simulink model "Sensitivity_Analysis"  (R2023a)
settings: Solver=VariableStepAuto  StartTime=0.0  StopTime=10.0  RelTol=1e-3
undefined symbols (not defined in the file or in its folder): Ion, Lithium
libraries: spsSeriesRLCBranchLib x84, spsControlledCurrentSourceLib x54, spsCurrentMeasurementLib x42, spsVoltageMeasurementLib x42, spsControlledVoltageSourceLib x18, spsBatteryLib x6, sps_lib x6
(part 1 of 6)
settings Model: Creator=40485811  LastModifiedBy=40485811

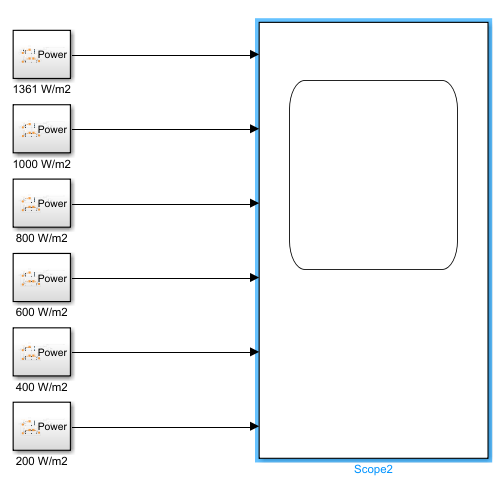
[thumbnail: Simulink's stored preview of the top-level diagram]
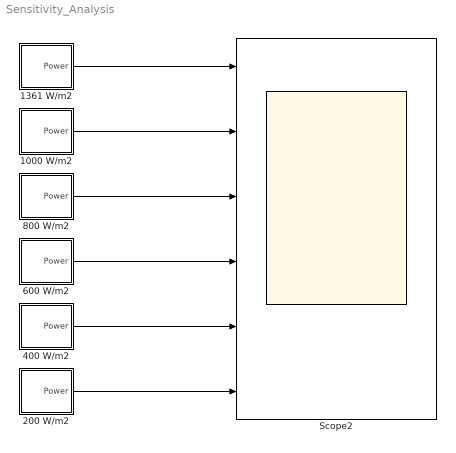
== system Sensitivity_Analysis ==
  1000 W/m2 : Subsystem
  1361 W/m2 : Subsystem
  200 W/m2 : Subsystem
  400 W/m2 : Subsystem
  600 W/m2 : Subsystem
  800 W/m2 : Subsystem
  Scope2 : Scope  NumInputPorts=6
  wires:
  1000 W/m2/1(Power) -> Scope2/2
  1361 W/m2/1(Power) -> Scope2/1
  800 W/m2/1(Power) -> Scope2/3
  600 W/m2/1(Power) -> Scope2/4
  200 W/m2/1(Power) -> Scope2/6
  400 W/m2/1(Power) -> Scope2/5

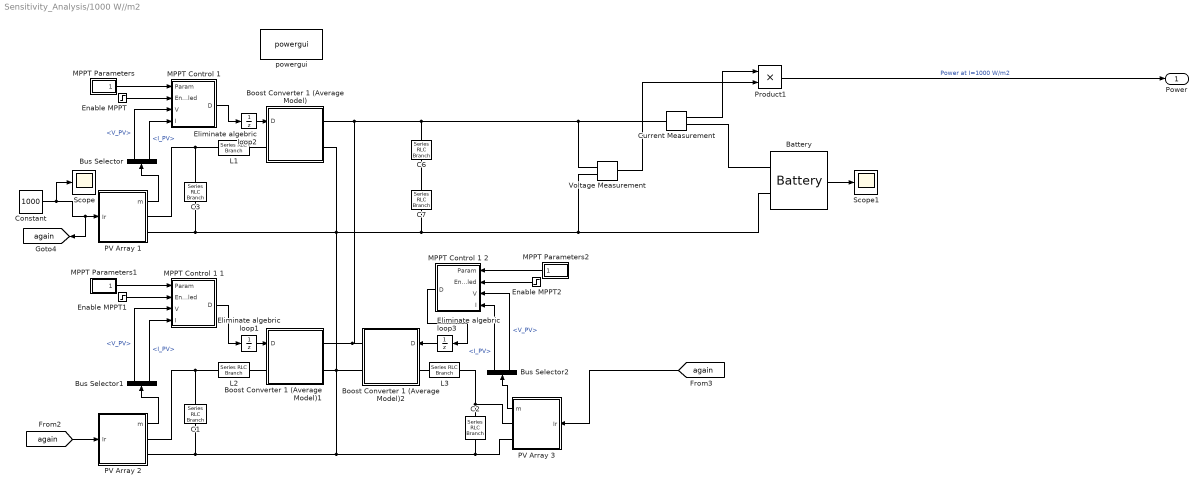
== system Sensitivity_Analysis/1000 W//m2 ==
  Battery : spsBatteryLib/Battery  BatType=Lithium-Ion  ShowTempParam=off  ThermalPreset=no  ShowAgeParam=off  NomV=7.2  NomQ=1000  SOC=100  Batt_Tr=30  PresetModel=on  MaxQ=1000  MinV=5.4  FullV=8.3807  Dis_rate=434.7826  R=7.2e-05  Normal_OP=904.3478  expZone="[7.77878      49.1304]"  current=[6.5 13 32.5]  Units=Time  Tci=20  NomT=20  T2=-30  MaxQ2=4.8  FullV2=7.1  Normal_OP2=5.655  expZone2="[6.58           1]"  Rca=0.6  ti=2000  Dp=0  Neq0=0  Tsim=1e6  Ta1=25  Qeol=5.4*0.9  Reol=0.013333*1.2  Char_age=[2.3478, 3]  Dis_age=[2.3478, 10]  N1=1500  N2=10500  N3=1000  N4=1400  Ta2=45  N5=950
  Boost Converter 1 (Average Model) : Subsystem  mask(Boost Converter (Average Model)){Ts=50e-6}
      mask prompts: Ts "Sample time:"
      mask Display: disp('Boost\n(Average)')
  Boost Converter 1 (Average Model)1 : Subsystem  mask(Boost Converter (Average Model)){Ts=50e-6}
      mask prompts: Ts "Sample time:"
      mask Display: disp('Boost\n(Average)')
  Boost Converter 1 (Average Model)2 : Subsystem  mask(Boost Converter (Average Model)){Ts=50e-6}
      mask prompts: Ts "Sample time:"
      mask Display: disp('Boost\n(Average)')
  Bus Selector : BusSelector  OutputSignals=V_PV,I_PV
  Bus Selector1 : BusSelector  OutputSignals=V_PV,I_PV
  Bus Selector2 : BusSelector  OutputSignals=V_PV,I_PV
  C1 : spsSeriesRLCBranchLib/Series RLC Branch  LConnTagsString=__new0  RConnTagsString=__new0  BranchType=C  Resistance=1.0  Inductance=1.0  SetiL0=off  InitialCurrent=0  Capacitance=100e-6  Setx0=off  InitialVoltage=0  Measurements=Branch voltage
  C2 : spsSeriesRLCBranchLib/Series RLC Branch  LConnTagsString=__new0  RConnTagsString=__new0  BranchType=C  Resistance=1.0  Inductance=1.0  SetiL0=off  InitialCurrent=0  Capacitance=100e-6  Setx0=off  InitialVoltage=0  Measurements=Branch voltage
  C3 : spsSeriesRLCBranchLib/Series RLC Branch  LConnTagsString=__new0  RConnTagsString=__new0  BranchType=C  Resistance=1.0  Inductance=1.0  SetiL0=off  InitialCurrent=0  Capacitance=100e-6  Setx0=off  InitialVoltage=0  Measurements=Branch voltage
  C6 : spsSeriesRLCBranchLib/Series RLC Branch  LConnTagsString=__new0  RConnTagsString=__new0  BranchType=C  Resistance=1.0  Inductance=1.0  SetiL0=off  InitialCurrent=0  Capacitance=24000e-06  Setx0=off  InitialVoltage=0  Measurements=None
  C7 : spsSeriesRLCBranchLib/Series RLC Branch  LConnTagsString=__new0  RConnTagsString=__new0  BranchType=C  Resistance=1.0  Inductance=1.0  SetiL0=off  InitialCurrent=0  Capacitance=24000e-06  Setx0=off  InitialVoltage=0  Measurements=None
  Constant : Constant  Value=1000
  Current Measurement : spsCurrentMeasurementLib/Current Measurement  PhasorSimulation=off  OutputType=Complex  PSBequivalent=0
  Eliminate algebric loop1 : UnitDelay  SampleTime=100e-6  HasFrameUpgradeWarning=on
  Eliminate algebric loop2 : UnitDelay  SampleTime=100e-6  HasFrameUpgradeWarning=on
  Eliminate algebric loop3 : UnitDelay  SampleTime=100e-6  HasFrameUpgradeWarning=on
  Enable MPPT : Step  Time=0.3  SampleTime=0
  Enable MPPT1 : Step  Time=0.3  SampleTime=0
  Enable MPPT2 : Step  Time=0.3  SampleTime=0
  L1 : spsSeriesRLCBranchLib/Series RLC Branch  LConnTagsString=__new0  RConnTagsString=__new0  BranchType=RL  Resistance=0.005  Inductance=5e-3  SetiL0=off  InitialCurrent=0  Capacitance=1e-6  Setx0=off  InitialVoltage=0  Measurements=None
  L2 : spsSeriesRLCBranchLib/Series RLC Branch  LConnTagsString=__new0  RConnTagsString=__new0  BranchType=RL  Resistance=0.005  Inductance=5e-3  SetiL0=off  InitialCurrent=0  Capacitance=1e-6  Setx0=off  InitialVoltage=0  Measurements=None
  L3 : spsSeriesRLCBranchLib/Series RLC Branch  LConnTagsString=__new0  RConnTagsString=__new0  BranchType=RL  Resistance=0.005  Inductance=5e-3  SetiL0=off  InitialCurrent=0  Capacitance=1e-6  Setx0=off  InitialVoltage=0  Measurements=None
  MPPT Parameters : Subsystem
  MPPT Parameters1 : Subsystem
  MPPT Parameters2 : Subsystem
  "MPPT Control 1 " : MATLAB Function  TreatAsAtomicUnit=on
  MPPT Control 1 1 : MATLAB Function  TreatAsAtomicUnit=on
  MPPT Control 1 2 : MATLAB Function  TreatAsAtomicUnit=on
  PV Array 1 : Subsystem  mask(PV array){ModuleType=SunPower SPR-305-WHT, Ncell=96, Nser=2500, Npar=2500, ModuleParameters=[ 64.2  5.96  54.7  5.58 ], ModelParameters=[ 0.037998  993.51  1.1753e-08  5.9602  1.3 ], Ts=50e-6, PlotVI_module=off, PlotVI_array=off}
      mask prompts: ModuleType "Module type:"; Ncell "Number of cells per module"; Nser "Number of series-connected  modules per string"; Npar "Number of parallel strings"; ModuleParameters "Module specifications under STC  [  Voc, Isc, Vmp, Imp ]"; ModelParameters "Model parameters for 1 module [ Rs, Rp, Isat, Iph, Qd ]"; Ts "Sample time"; PlotVI_module "Display  I-V and  P-V characteritics of one module"; PlotVI_array "Display  I-V and  P-V characteritics of array"
      mask help:
      | Model a PV array
      |
      | PV array consists of Npar strings of modules connected in parallel, each string consisting of Nser modules connected in series.
      |
      | The four PV model parameters (photo-generated current Iph, diode saturation current Isat, parallel resistance Rp and  series resistance Rs) are adjuted to fit the following four module characteristics measured under standard test conditions (STC : irradiance 1000 W/m^2, cell temperature=25 deg. C) and assuming a given "diode quality factor" (Qd) for the semiconductor:
      |   Voc = open circuit voltage
      |   Isc = short-circuit current
      |   Vmp,Imp = voltage and current at maximum power point
      |
      | Select a 'Module type' and then press Apply to see module parameters.
      | Note: Module characteristics are extracted from NREL System Advisor Model.
      mask init:
      | BlockName=gcb;
      | 
      | % SolarModuleSpec_Definition_v2.m
      | %================================
      | %
      | Type=1;
      | SolarModuleSpec(Type).Desc= 'Kyocera KD135GX-LP';
      | SolarModuleSpec(Type).nCells= 36;              % Number of cells in series
      | SolarModuleSpec(Type).Pmp= 135.044;            % Maximum power (W)
      | SolarModuleSpec(Type).Vmp= 17.7;               % Maximum power voltage (V) 
      | SolarModuleSpec(Type).Imp= 7.62959;            % Maximum power current (A)
      | SolarModuleSpec(Type).Voc= 22.0999;            % Open circuit voltage (V)
      | SolarModuleSpec(Type).Isc= 8.36955;            % Short circuit current (A)
      | SolarModuleSpec(Type).TempC_Pmp= -6.445e-001;  % Maximum power temp. coefficient (W/deg.C)
      | SolarModuleSpec(Type).TempC_Vmp= -8.200e-002;  % Maximum power voltage temp. coefficient (V/deg.C)
      | SolarModuleSpec(Type).TempC_Imp= -1.068e-003;  % Maximum power current temp. coefficient (A/deg.C
      | SolarModuleSpec(Type).TempC_Voc= -8.000e-002;  % Open circuit voltage temp. coefficient (V/deg.C)
      | SolarModuleSpec(Type).TempC_Isc= 5.022e-003;   % Short circuit current temp. coefficient (A/deg.C)
      | SolarModuleSpec(Type).Rs= 0.10593;             % Series resistance of PV model (ohms)
      | SolarModuleSpec(Type).Rp= 142.84;              % Parallel resistance of PV model (ohms)
      | SolarModuleSpec(Type).Isat= 9.845e-07;         % Diode saturation current of PV model (A)
      | SolarModuleSpec(Type).Iph=  8.3758;            % Light-generated photo-current  of PV model (A)
      | SolarModuleSpec(Type).Qd= 1.5;                 % Diode quality factor of PV model
      | %-------------------------------------------------------------------------
      | %
      | Type=2;
      | SolarModuleSpec(Type).Desc= 'Kyocera KD205GX-LP';
      | SolarModuleSpec(Type).nCells= 54;              % Number of cells in series
      | SolarModuleSpec(Type).Pmp= 205.075;            % Maximum power (W)
      | SolarModuleSpec(Type).Vmp= 26.6;               % Maximum power voltage (V) 
      | SolarModuleSpec(Type).Imp= 7.70959;            % Maximum power current (A)
      | SolarModuleSpec(Type).Voc= 33.1999;            % Open circuit voltage (V)
      | SolarModuleSpec(Type).Isc= 8.35955;            % Short circuit current (A)
      | SolarModuleSpec(Type).TempC_Pmp= -9.770e-001;  % Maximum power temp. coefficient (W/deg.C)
      | SolarModuleSpec(Type).TempC_Vmp= -1.230e-001;  % Maximum power voltage temp. coefficient (V/deg.C)
      | SolarModuleSpec(Type).TempC_Imp= -1.079e-003;  % Maximum power current temp. coefficient (A/deg.C
      | SolarModuleSpec(Type).TempC_Voc= -1.200e-001;  % Open circuit voltage temp. coefficient (V/deg.C)
      | SolarModuleSpec(Type).TempC_Isc= 5.016e-003;   % Short circuit current temp. coefficient (A/deg.C)
      | SolarModuleSpec(Type).Rs= 0.15945;             % Series resistance of PV model (ohms)
      | SolarModuleSpec(Type).Rp= 1010.6;              % Parallel resistance of PV model (ohms)
      | SolarModuleSpec(Type).Isat=  9.7399e-07;       % Diode saturation current of PV model (A)
      | SolarModuleSpec(Type).Iph= 8.3642;             % Light-generated photo-current  of PV model (A)
      | SolarModuleSpec(Type).Qd= 1.5;                 % Diode quality factor of PV model
      | %-------------------------------------------------------------------------
      | %
      | Type=3;
      | SolarModuleSpec(Type).Desc= 'Mitsubishi PV-UD190MF5';
      | SolarModuleSpec(Type).nCells= 50;              % Number of cells in series
      | SolarModuleSpec(Type).Pmp= 190.503;            % Maximum power (W)
      | SolarModuleSpec(Type).Vmp= 24.6999;            % Maximum power voltage (V) 
      | SolarModuleSpec(Type).Imp= 7.71272;            % Maximum power current (A)
      | SolarModuleSpec(Type).Voc= 30.8006;            % Open circuit voltage (V)
      | SolarModuleSpec(Type).Isc= 8.23289;            % Short circuit current (A)
      | SolarModuleSpec(Type).TempC_Pmp= -8.597e-001;  % Maximum power temp. coefficient (W/deg.C)
      | SolarModuleSpec(Type).TempC_Vmp= -1.090e-001;  % Maximum power voltage temp. coefficient (V/deg.C)
      | SolarModuleSpec(Type).TempC_Imp= -7.713e-004;  % Maximum power current temp. coefficient (A/deg.C
      | SolarModuleSpec(Type).TempC_Voc= -1.050e-001;  % Open circuit voltage temp. coefficient (V/deg.C)
      | SolarModuleSpec(Type).TempC_Isc= 4.446e-003;   % Short circuit current temp. coefficient (A/deg.C)
      | SolarModuleSpec(Type).Rs= 0.20758;             % Series resistance of PV model (ohms)
      | SolarModuleSpec(Type).Rp= 975.6;               % Parallel resistance of PV model (ohms)
      | SolarModuleSpec(Type).Isat= 7.9676e-08;        % Diode saturation current of PV model (A)
      | SolarModuleSpec(Type).Iph= 8.2649;             % Light-generated photo-current  of PV model (A)
      | SolarModuleSpec(Type).Qd= 1.3;                 % Diode quality factor of PV model
      | %-------------------------------------------------------------------------
      | %
      | Type=4;
      | SolarModuleSpec(Type).Desc= 'Sanyo HIP-225HDE1';
      | SolarModuleSpec(Type).nCells= 60;              % Number of cells in series
      | SolarModuleSpec(Type).Pmp= 224.899;            % Maximum power (W)
      | SolarModuleSpec(Type).Vmp= 33.9;               % Maximum power voltage (V) 
      | SolarModuleSpec(Type).Imp= 6.63419;            % Maximum power current (A)
      | SolarModuleSpec(Type).Voc= 41.7984;            % Open circuit voltage (V)
      | SolarModuleSpec(Type).Isc= 7.13383;            % Short circuit current (A)
      | SolarModuleSpec(Type).TempC_Pmp= -6.925e-001;  % Maximum power temp. coefficient (W/deg.C)
      | SolarModuleSpec(Type).TempC_Vmp= -1.010e-001;  % Maximum power voltage temp. coefficient (V/deg.C)
      | SolarModuleSpec(Type).TempC_Imp= -6.634e-004;  % Maximum power current temp. coefficient (A/deg.C
      | SolarModuleSpec(Type).TempC_Voc= -1.050e-001;  % Open circuit voltage temp. coefficient (V/deg.C)
      | SolarModuleSpec(Type).TempC_Isc= 2.140e-003;   % Short circuit current temp. coefficient (A/deg.C)
      | SolarModuleSpec(Type).Rs=  0.20439;            % Series resistance of PV model (ohms)
      | SolarModuleSpec(Type).Rp= 1830.7;              % Parallel resistance of PV model (ohms)
      | SolarModuleSpec(Type).Isat=  3.0815e-07;       % Diode saturation current of PV model (A)
      | SolarModuleSpec(Type).Iph=  7.145;             % Light-generated photo-current  of PV model (A)
      | SolarModuleSpec(Type).Qd= 1.6;                 % Diode quality factor of PV model
      | %-------------------------------------------------------------------------
      | %
      | 
      | Type=5;
      | % NREL : 2007(E)
      | SolarModuleSpec(Type).Desc= 'SunPower SPR-305-WHT';
      | SolarModuleSpec(Type).nCells= 96;              % Number of cells in series
      | SolarModuleSpec(Type).Pmp= 305.2;              % Maximum power (W)
      | SolarModuleSpec(Type).Vmp= 54.70;              % Maximum power voltage (V) 
      | SolarModuleSpec(Type).Imp= 5.58;               % Maximum power current (A)
      | SolarModuleSpec(Type).Voc= 64.20;              % Open circuit voltage (V)
      | SolarModuleSpec(Type).Isc= 5.96;               % Short circuit current (A)
      | SolarModuleSpec(Type).TempC_Pmp= -1.154e+000;  % Maximum power temp. coefficient (W/deg.C)
      | SolarModuleSpec(Type).TempC_Vmp= -1.860e-001;  % Maximum power voltage temp. coefficient (V/deg.C)
      | SolarModuleSpec(Type).TempC_Imp= -2.120e-003;  % Maximum power current temp. coefficient (A/deg.C
      | SolarModuleSpec(Type).TempC_Voc= -1.770e-001;  % Open circuit voltage temp. coefficient (V/deg.C)
      | SolarModuleSpec(Type).TempC_Isc= 3.516e-003;   % Short circuit current temp. coefficient (A/deg.C)
      | SolarModuleSpec(Type).Rs= 0.037998;            % Series resistance of PV model (ohms)
      | SolarModuleSpec(Type).Rp= 993.51;              % Parallel resistance of PV model (ohms)
      | SolarModuleSpec(Type).Isat= 1.1753e-08;        % Diode saturation current of PV model (A)
      | SolarModuleSpec(Type).Iph= 5.9602;             % Light-generated photo-current  of PV model (A)
      | SolarModuleSpec(Type).Qd= 1.3;                 % Diode quality factor of PV model
      | %-------------------------------------------------------------------------
      | %
      | Type=6;
      | SolarModuleSpec(Type).Desc= 'Suntech STP270S-24_Vb';
      | SolarModuleSpec(Type).nCells= 72;              % Number of cells in series
      | SolarModuleSpec(Type).Pmp= 269.843;            % Maximum power (W)
      | SolarModuleSpec(Type).Vmp= 35;                 % Maximum power voltage (V) 
      | SolarModuleSpec(Type).Imp= 7.70979;            % Maximum power current (A)
      | SolarModuleSpec(Type).Voc= 44.4999;            % Open circuit voltage (V)
      | SolarModuleSpec(Type).Isc= 8.19978;            % Short circuit current (A)
      | SolarModuleSpec(Type).TempC_Pmp= -1.204e+000;  % Maximum power temp. coefficient (W/deg.C)
      | SolarModuleSpec(Type).TempC_Vmp= -1.567e-001;  % Maximum power voltage temp. coefficient (V/deg.C)
      | SolarModuleSpec(Type).TempC_Imp= 1.234e-004;   % Maximum power current temp. coefficient (A/deg.C
      | SolarModuleSpec(Type).TempC_Voc= -1.504e-001;  % Open circuit voltage temp. coefficient (V/deg.C)
      | SolarModuleSpec(Type).TempC_Isc= 4.969e-003;   % Short circuit current temp. coefficient (A/deg.C)
      | SolarModuleSpec(Type).Rs= 0.32025;             % Series resistance of PV model (ohms)
      | SolarModuleSpec(Type).Rp= 2562.3;              % Parallel resistance of PV model (ohms)
      | SolarModuleSpec(Type).Isat= 8.8992e-07;        % Diode saturation current of PV model (A)
      | SolarModuleSpec(Type).Iph= 8.2979;             % Light-generated photo-current  of PV model (A)
      | SolarModuleSpec(Type).Qd= 1.5;                 % Diode quality factor of PV model
      | % 
      | %-------------------------------------------------------------------------
      | %
      | Type=7;
      | SolarModuleSpec(Type).Desc= 'Canadian Solar CS5P-220M';
      | SolarModuleSpec(Type).nCells= 96;              % Number of cells in series
      | SolarModuleSpec(Type).Pmp= 219.72;             % Maximum power (W)
      | SolarModuleSpec(Type).Vmp= 48.3159;            % Maximum power voltage (V) 
      | SolarModuleSpec(Type).Imp= 4.54758;            % Maximum power current (A)
      | SolarModuleSpec(Type).Voc= 59.2618;            % Open circuit voltage (V)
      | SolarModuleSpec(Type).Isc= 5.09261;            % Short circuit current (A)
      | SolarModuleSpec(Type).TempC_Pmp= -1.031e+000;  % Maximum power temp. coefficient (W/deg.C)
      | SolarModuleSpec(Type).TempC_Vmp= -2.355e-001;  % Maximum power voltage temp. coefficient (V/deg.C)
      | SolarModuleSpec(Type).TempC_Imp= 8.231e-004;   % Maximum power current temp. coefficient (A/deg.C
      | SolarModuleSpec(Type).TempC_Voc= -2.170e-001;  % Open circuit voltage temp. coefficient (V/deg.C)
      | SolarModuleSpec(Type).TempC_Isc= 2.022e-003;   % Short circuit current temp. coefficient (A/deg.C)
      | SolarModuleSpec(Type).Rs= 0.24807;             % Series resistance of PV model (ohms)
      | SolarModuleSpec(Type).Rp= 235.76;              % Parallel resistance of PV model (ohms)
      | SolarModuleSpec(Type).Isat= 5.3103e-07;        % Diode saturation current of PV model (A)
      | SolarModuleSpec(Type).Iph= 5.098;              % Light-generated photo-current  of PV model (A)
      | SolarModuleSpec(Type).Qd= 1.5;                 % Diode quality factor of PV model
      | %-------------------------------------------------------------------------
      | %
      | Type=8;
      | SolarModuleSpec(Type).Desc= 'BP Solar SX3190';
      | SolarModuleSpec(Type).nCells= 50;              % Number of cells in series
      | SolarModuleSpec(Type).Pmp= 190.258;            % Maximum power (W)
      | SolarModuleSpec(Type).Vmp= 24.3003;            % Maximum power voltage (V) 
      | SolarModuleSpec(Type).Imp= 7.82945;            % Maximum power current (A)
      | SolarModuleSpec(Type).Voc= 30.6021;            % Open circuit voltage (V)
      | SolarModuleSpec(Type).Isc= 8.51029;            % Short circuit current (A)
      | SolarModuleSpec(Type).TempC_Pmp= -9.306e-001;  % Maximum power temp. coefficient (W/deg.C)
      | SolarModuleSpec(Type).TempC_Vmp= -1.140e-001;  % Maximum power voltage temp. coefficient (V/deg.C)
      | SolarModuleSpec(Type).TempC_Imp= -1.566e-003;  % Maximum power current temp. coefficient (A/deg.C
      | SolarModuleSpec(Type).TempC_Voc= -1.110e-001;  % Open circuit voltage temp. coefficient (V/deg.C)
      | SolarModuleSpec(Type).TempC_Isc= 5.532e-003;   % Short circuit current temp. coefficient (A/deg.C)
      | SolarModuleSpec(Type).Rs= 0.17514;             % Series resistance of PV model (ohms)
      | SolarModuleSpec(Type).Rp= 755.51;              % Parallel resistance of PV model (ohms)
      | SolarModuleSpec(Type).Isat= 1.0647e-06;       % Diode saturation current of PV model (A)
      | SolarModuleSpec(Type).Iph= 8.5158;             % Light-generated photo-current  of PV model (A)
      | SolarModuleSpec(Type).Qd= 1.5;                 % Diode quality factor of PV model
      | %-------------------------------------------------------------------------
      | %
      | Type=9;
      | SolarModuleSpec(Type).Desc= 'First Solar FS-272';
      | SolarModuleSpec(Type).nCells= 116;             % Number of cells in series
      | SolarModuleSpec(Type).Pmp= 71.326;             % Maximum power (W)
      | SolarModuleSpec(Type).Vmp= 70.558;             % Maximum power voltage (V) 
      | SolarModuleSpec(Type).Imp= 1.01088;            % Maximum power current (A)
      | SolarModuleSpec(Type).Voc= 94.5738;            % Open circuit voltage (V)
      | SolarModuleSpec(Type).Isc= 1.18103;            % Short circuit current (A)
      | SolarModuleSpec(Type).TempC_Pmp= -2.332e-001;  % Maximum power temp. coefficient (W/deg.C)
      | SolarModuleSpec(Type).TempC_Vmp= -2.060e-001;  % Maximum power voltage temp. coefficient (V/deg.C)
      | SolarModuleSpec(Type).TempC_Imp= -3.538e-004;  % Maximum power current temp. coefficient (A/deg.C
      | SolarModuleSpec(Type).TempC_Voc= -2.690e-001;  % Open circuit voltage temp. coefficient (V/deg.C)
      | SolarModuleSpec(Type).TempC_Isc= 5.433e-004;   % Short circuit current temp. coefficient (A/deg.C)
      | SolarModuleSpec(Type).Rs= 7.7692;              % Series resistance of PV model (ohms)
      | SolarModuleSpec(Type).Rp= 1044.9;              % Parallel resistance of PV model (ohms)
      | SolarModuleSpec(Type).Isat= 1.1116e-068;       % Diode saturation current of PV model (A)
      | SolarModuleSpec(Type).Iph= 1.1898;             % Light-generated photo-current  of PV model (A)
      | SolarModuleSpec(Type).Qd= 2.3;                 % Diode quality factor of PV model
      | %-------------------------------------------------------------------------
      | %
      | Type=10;
      | SolarModuleSpec(Type).Desc= 'SunPower 128-cell Module';
      | SolarModuleSpec(Type).nCells= 128;             % Number of cells in series
      | SolarModuleSpec(Type).Pmp= 400.048;            % Maximum power (W)
      | SolarModuleSpec(Type).Vmp= 72.8992;            % Maximum power voltage (V) 
      | SolarModuleSpec(Type).Imp= 5.48769;            % Maximum power current (A)
      | SolarModuleSpec(Type).Voc= 85.2983;            % Open circuit voltage (V)
      | SolarModuleSpec(Type).Isc= 5.8675;             % Short circuit current (A)
      | SolarModuleSpec(Type).TempC_Pmp= -1.638e+000;  % Maximum power temp. coefficient (W/deg.C)
      | SolarModuleSpec(Type).TempC_Vmp= -2.760e-001;  % Maximum power voltage temp. coefficient (V/deg.C)
      | SolarModuleSpec(Type).TempC_Imp= -1.690e-003;  % Maximum power current temp. coefficient (A/deg.C
      | SolarModuleSpec(Type).TempC_Voc= -2.664e-001;  % Open circuit voltage temp. coefficient (V/deg.C)
      | SolarModuleSpec(Type).TempC_Isc= 1.837e-003;   % Short circuit current temp. coefficient (A/deg.C)
      | SolarModuleSpec(Type).Rs= 0.12264;             % Series resistance of PV model (ohms)
      | SolarModuleSpec(Type).Rp= 859.93;              % Parallel resistance of PV model (ohms)
      | SolarModuleSpec(Type).Isat= 2.3385e-09;        % Diode saturation current of PV model (A)
      | SolarModuleSpec(Type).Iph= 5.8683;             % Light-generated photo-current  of PV model (A)
      | SolarModuleSpec(Type).Qd= 1.2;                 % Diode quality factor of PV model
      | %-------------------------------------------------------------------------
      | 
      | Type=strmatch(ModuleType,char(SolarModuleSpec.Desc));
      | 
      | k= 1.3806e-23; % Boltzman constant (J.K^-1)
      | q=1.6022e-19;  % electron charge  (C)
      | T=273+25;
      | 
      | nCells=SolarModuleSpec(Type).nCells;
      | Voc=SolarModuleSpec(Type).Voc;
      | Isc=SolarModuleSpec(Type).Isc;
      | Vm=SolarModuleSpec(Type).Vmp;
      | Im=SolarModuleSpec(Type).Imp;
      | 
      | set_param(BlockName,'Ncell',num2str(nCells));
      | str=sprintf('[ %g  %g  %g  %g ]',Voc,Isc,Vm,Im);
      | set_param(BlockName,'ModuleParameters',str);
      | 
      | Rs=SolarModuleSpec(Type).Rs;
      | Rp=SolarModuleSpec(Type).Rp; 
      | Isat=SolarModuleSpec(Type).Isat;
      | Iph=SolarModuleSpec(Type).Iph;            
      | Qd=SolarModuleSpec(Type).Qd;
      | 
      | VT=k*T/q*nCells*Qd;
      | 
      | str=sprintf('[ %g  %g  %g  %g  %g ]',Rs,Rp,Isat,Iph, Qd);
      | set_param(BlockName,'ModelParameters',str)
      | 
      | Iph_array=Iph*Npar;
      | Isat_array=Isat*Npar;
      | VT_array=VT*Nser;
      | Rs_array=Rs*Nser/Npar;
      | Rp_array=Rp*Nser/Npar;
      | %
      | %% Plot I-V & P-V characteristics of one module
      | %==============================================
      | if PlotVI_module | PlotVI_array
      |     assignin('base','Voc',Voc);
      |     assignin('base','Isc',Isc);
      |     assignin('base','Rs',Rs);
      |     assignin('base','Rp',Rp);
      |     assignin('base','Isat',Isat);
      |     assignin('base','VT',VT);
      |      
      |     if PlotVI_module, 
      |         F1=figure('Name','I-V and P-V characteristics of one module at 25 deg.C');
      |     end
      |     if PlotVI_array ,
      |         F2=figure('Name','I-V and P-V characteristics of array at 25 deg.C');  
      |     end
      |     load_system('PV_model_Param');
      |     
      |     for ksun=1:-0.25:0.25
      |         assignin('base','Iph',Iph*ksun)
      |         sim('PV_model_Param');
      |         n=find(I_PV>=0);
      |         I_PV=I_PV(n);
      |         V_PV=V_PV(n);
      |         P_PV=V_PV.*I_PV;
      |         
      |         if PlotVI_module
      |             figure(F1);
      |             subplot(211)
      |             if ksun==1
      |                 plot(V_PV,I_PV,'b',[0  Vm Voc], [Isc Im 0],'ro')
      |                 text(Voc/15,Isc*1.1,'1 kW/m^2')
      |                 hold on
      |                 grid
      |             else
      |                 plot(V_PV,I_PV,'--m')
      |                 text(Voc/15, Isc*(ksun+0.1) , sprintf('%g kW/m^2',ksun))
      |             end
      | 
      |             subplot(212) 
      |             if ksun==1
      |                 plot(V_PV,P_PV,'b',[0  Vm Voc], [0 Im*Vm 0],'ro')
      |                 text(Vm*1.02,Vm*Im,'1 kW/m^2')
      |                 hold on
      |                 grid
      |             else
      |                 n= find(P_PV==max(P_PV));
      |                 plot(V_PV,P_PV,'--m', V_PV(n) , P_PV(n),'mo')
      |                 text(Vm*1.02, Vm*Im*ksun, sprintf('%g kW/m^2',ksun))
      |             end
      |             subplot(211)
      |             ylabel('Current (A)')
      |             xlabel('Voltage (V)')
      |             title(sprintf('Module type: %s',SolarModuleSpec(Type).Desc))
      |             axis_xy=axis;
      |             axis_xy(4)=Isc*1.2;
      |             axis(axis_xy);
      |             
      |             subplot(212)
      |             ylabel('Power (W)')
      |             xlabel('Voltage (V)')
      |             axis_xy=axis;
      |             axis_xy(4)=Vm*Im*1.2;
      |             axis(axis_xy);
      |                   
      |             set_param(BlockName,'PlotVI_module', 'off')
      |         end
      |         
      |         if PlotVI_array
      |             figure(F2);
      |             subplot(211)
      |             if ksun==1
      |                 plot(V_PV*Nser,I_PV*Npar,'b',[0  Vm Voc]*Nser, [Isc Im 0]*Npar,'ro')
      |                 text(Voc/15*Nser,Isc*1.1*Npar,'1 kW/m^2')
      |                 hold on
      |                 grid
      |             else
      |                 plot(V_PV*Nser,I_PV*Npar,'--m')
      |                 text(Voc*Nser/15, Isc*Npar*(ksun+0.1) , sprintf('%g kW/m^2',ksun))
      |             end
      |            
      | 
      |             subplot(212)
      |             if ksun==1
      |                 plot(V_PV*Nser,P_PV*Nser*Npar,'b',[0  Vm Voc]*Nser, [0 Im*Vm 0]*Nser*Npar,'ro')
      |                 text(Vm*Nser*1.02,Vm*Im*Nser*Npar,'1 kW/m^2')
      |                 hold on
      |                 grid
      |             else
      |                 n= find(P_PV==max(P_PV));
      |                 plot(V_PV*Nser,P_PV*Nser*Npar,'--m', V_PV(n)*Nser , P_PV(n)*Nser*Npar,'mo')
      |                 text(Vm*Nser*1.02, Vm*Im*Nser*Npar*ksun, sprintf('%g kW/m^2',ksun))
      |             end 
      |             subplot(211)
      |             ylabel('Current (A)')
      |             xlabel('Voltage (V)')
      |             title(sprintf('Array type: %s; %d series modules; %d parallel strings',SolarModuleSpec(Type).Desc,Nser,Npar));
      |             axis_xy=axis;
      |             axis_xy(4)=Isc*Npar*1.2;
      |             axis(axis_xy);
      |             
      |             subplot(212)
      |             ylabel('Power (W)')
      |             xlabel('Voltage (V)')
      |             xis_xy=axis;
      |             axis_xy(4)=Vm*Im*Nser*Npar*1.2;
      |             axis(axis_xy);
      |             
      |             set_param(BlockName,'PlotVI_array', 'off')
      |         end
      |         
      |     end  
      | end
      mask TypeOptions ModuleType: BP Solar SX3190 | Canadian Solar CS5P-220M | First Solar FS-272 | Kyocera KD135GX-LP | Kyocera KD205GX-LP | Mitsubishi PV-UD190MF5 | Sanyo HIP-225HDE1 | SunPower SPR-305-WHT | SunPower SPR-400-WHT | Suntech STP270S-24_Vb
      mask Display: image(imread('panel.jpg'))
  PV Array 2 : Subsystem  mask(PV array){ModuleType=SunPower SPR-305-WHT, Ncell=96, Nser=2500, Npar=2500, ModuleParameters=[ 64.2  5.96  54.7  5.58 ], ModelParameters=[ 0.037998  993.51  1.1753e-08  5.9602  1.3 ], Ts=50e-6, PlotVI_module=off, PlotVI_array=off}
      mask prompts: ModuleType "Module type:"; Ncell "Number of cells per module"; Nser "Number of series-connected  modules per string"; Npar "Number of parallel strings"; ModuleParameters "Module specifications under STC  [  Voc, Isc, Vmp, Imp ]"; ModelParameters "Model parameters for 1 module [ Rs, Rp, Isat, Iph, Qd ]"; Ts "Sample time"; PlotVI_module "Display  I-V and  P-V characteritics of one module"; PlotVI_array "Display  I-V and  P-V characteritics of array"
      mask help:
      | Model a PV array
      |
      | PV array consists of Npar strings of modules connected in parallel, each string consisting of Nser modules connected in series.
      |
      | The four PV model parameters (photo-generated current Iph, diode saturation current Isat, parallel resistance Rp and  series resistance Rs) are adjuted to fit the following four module characteristics measured under standard test conditions (STC : irradiance 1000 W/m^2, cell temperature=25 deg. C) and assuming a given "diode quality factor" (Qd) for the semiconductor:
      |   Voc = open circuit voltage
      |   Isc = short-circuit current
      |   Vmp,Imp = voltage and current at maximum power point
      |
      | Select a 'Module type' and then press Apply to see module parameters.
      | Note: Module characteristics are extracted from NREL System Advisor Model.
      mask init: same as Sensitivity_Analysis/1000 W//m2/PV Array 1
      mask TypeOptions ModuleType: BP Solar SX3190 | Canadian Solar CS5P-220M | First Solar FS-272 | Kyocera KD135GX-LP | Kyocera KD205GX-LP | Mitsubishi PV-UD190MF5 | Sanyo HIP-225HDE1 | SunPower SPR-305-WHT | SunPower SPR-400-WHT | Suntech STP270S-24_Vb
      mask Display: image(imread('panel.jpg'))
  PV Array 3 : Subsystem  mask(PV array){ModuleType=SunPower SPR-305-WHT, Ncell=96, Nser=2500, Npar=2500, ModuleParameters=[ 64.2  5.96  54.7  5.58 ], ModelParameters=[ 0.037998  993.51  1.1753e-08  5.9602  1.3 ], Ts=50e-6, PlotVI_module=off, PlotVI_array=off}
      mask prompts: ModuleType "Module type:"; Ncell "Number of cells per module"; Nser "Number of series-connected  modules per string"; Npar "Number of parallel strings"; ModuleParameters "Module specifications under STC  [  Voc, Isc, Vmp, Imp ]"; ModelParameters "Model parameters for 1 module [ Rs, Rp, Isat, Iph, Qd ]"; Ts "Sample time"; PlotVI_module "Display  I-V and  P-V characteritics of one module"; PlotVI_array "Display  I-V and  P-V characteritics of array"
      mask help:
      | Model a PV array
      |
      | PV array consists of Npar strings of modules connected in parallel, each string consisting of Nser modules connected in series.
      |
      | The four PV model parameters (photo-generated current Iph, diode saturation current Isat, parallel resistance Rp and  series resistance Rs) are adjuted to fit the following four module characteristics measured under standard test conditions (STC : irradiance 1000 W/m^2, cell temperature=25 deg. C) and assuming a given "diode quality factor" (Qd) for the semiconductor:
      |   Voc = open circuit voltage
      |   Isc = short-circuit current
      |   Vmp,Imp = voltage and current at maximum power point
      |
      | Select a 'Module type' and then press Apply to see module parameters.
      | Note: Module characteristics are extracted from NREL System Advisor Model.
      mask init: same as Sensitivity_Analysis/1000 W//m2/PV Array 1
      mask TypeOptions ModuleType: BP Solar SX3190 | Canadian Solar CS5P-220M | First Solar FS-272 | Kyocera KD135GX-LP | Kyocera KD205GX-LP | Mitsubishi PV-UD190MF5 | Sanyo HIP-225HDE1 | SunPower SPR-305-WHT | SunPower SPR-400-WHT | Suntech STP270S-24_Vb
      mask Display: image(imread('panel.jpg'))
  Product1 : Product
  Scope : Scope
  Scope1 : Scope
  Voltage Measurement : spsVoltageMeasurementLib/Voltage Measurement  PhasorSimulation=off  OutputType=Complex  PSBequivalent=0
  powergui : sps_lib/powergui  Priority=1  SimulationMode=Continuous  SampleTime=50e-6  frequency=60  Iterations=50  frequencyindice=0  Pbase=100e6  ErrMax=1e-4  UnitsV=kV  UnitsW=MW  buscounter=0  FunctionMessages=off  echomessages=off  EnableUseOfTLC=off  CurrentSourceSwitches=off  DisableSnubberDevices=off  DisableRonSwitches=off  DisableVfSwitches=off  DisplayEquations=off  AutomaticDiscreteSolvers=off  SolverType=Tustin/Backward Euler (TBE)  Interpol=off  ExternalGateDelay=off  methode=off  Ts=100  x0status=blocks  SPID=on  SwTol=0  HookPort=off  NonlinearTolerance=1e-4  nMaxIteration=100  ContinueOnMaxIteration=off  RestoreLinks=warning  ResistiveCurrentMeasurement=off  Frange=[0:2:500]  Ylog=off  Xlog=on  ShowGrid=off  save=off  variable=ZData  structure=0  ZoomFFT=off  StartTime=0.0  cycles=1  DisplayStyle=1  fundamental=60  FreqAxis=off  MaxFrequency=1000  frequencyindicesteady=1  RmsSteady=1  display=off
  Power : Outport
  tag scope: again=global
  wires:
  Constant/1 -> PV Array 1/1(Ir), [again], Scope/1
  Bus Selector1/1 -> MPPT Control 1 1/3(V)  "<V_PV>"
  Enable MPPT/1 -> "MPPT Control 1 "/2(Enabled)
  Enable MPPT2/1 -> MPPT Control 1 2/2(Enabled)
  Eliminate algebric loop1/1 -> Boost Converter 1 (Average Model)1/1(D)
  Bus Selector1/2 -> MPPT Control 1 1/4(I)  "<I_PV>"
  Bus Selector2/2 -> MPPT Control 1 2/4(I)  "<I_PV>"
  Bus Selector/2 -> "MPPT Control 1 "/4(I)  "<I_PV>"
  PV Array 1/1(m) -> Bus Selector/1
  MPPT Parameters2/1(Param) -> MPPT Control 1 2/1(Param)
  "MPPT Control 1 "/1(D) -> Eliminate algebric loop2/1
  Product1/1 -> Power/1  "Power at I=1000 W/m2"
  Bus Selector/1 -> "MPPT Control 1 "/3(V)  "<V_PV>"
  Enable MPPT1/1 -> MPPT Control 1 1/2(Enabled)
  MPPT Parameters1/1(Param) -> MPPT Control 1 1/1(Param)
  [again] -> PV Array 2/1(Ir)
  PV Array 3/1(m) -> Bus Selector2/1
  MPPT Control 1 2/1(D) -> Eliminate algebric loop3/1
  MPPT Parameters/1(Param) -> "MPPT Control 1 "/1(Param)
  Eliminate algebric loop3/1 -> Boost Converter 1 (Average Model)2/1(D)
  Bus Selector2/1 -> MPPT Control 1 2/3(V)  "<V_PV>"
  MPPT Control 1 1/1(D) -> Eliminate algebric loop1/1
  [again] -> PV Array 3/1(Ir)
  PV Array 2/1(m) -> Bus Selector1/1
  Eliminate algebric loop2/1 -> Boost Converter 1 (Average Model)/1(D)
  Battery/1 -> Scope1/1
  Current Measurement/1 -> Product1/1
  Voltage Measurement/1 -> Product1/2
  connections:
  Current Measurement/RConn1 -- Battery/LConn1
  L3/LConn1 -- C2/LConn1 -- PV Array 3/RConn1
  C6/LConn1 -- Boost Converter 1 (Average Model)/RConn1 -- Boost Converter 1 (Average Model)2/RConn1 -- Boost Converter 1 (Average Model)1/RConn1 -- Voltage Measurement/LConn1 -- Current Measurement/LConn1
  L1/RConn1 -- Boost Converter 1 (Average Model)/LConn1
  C2/RConn1 -- PV Array 3/RConn2 -- Boost Converter 1 (Average Model)2/RConn2 -- Boost Converter 1 (Average Model)1/RConn2 -- Voltage Measurement/LConn2 -- Battery/LConn2 -- C7/RConn1 -- Boost Converter 1 (Average Model)/RConn2 -- PV Array 1/RConn2 -- C3/RConn1 -- PV Array 2/RConn2 -- C1/RConn1
  L1/LConn1 -- C3/LConn1 -- PV Array 1/RConn1
  L2/RConn1 -- Boost Converter 1 (Average Model)1/LConn1
  C6/RConn1 -- C7/LConn1
  C1/LConn1 -- L2/LConn1 -- PV Array 2/RConn1
  L3/RConn1 -- Boost Converter 1 (Average Model)2/LConn1

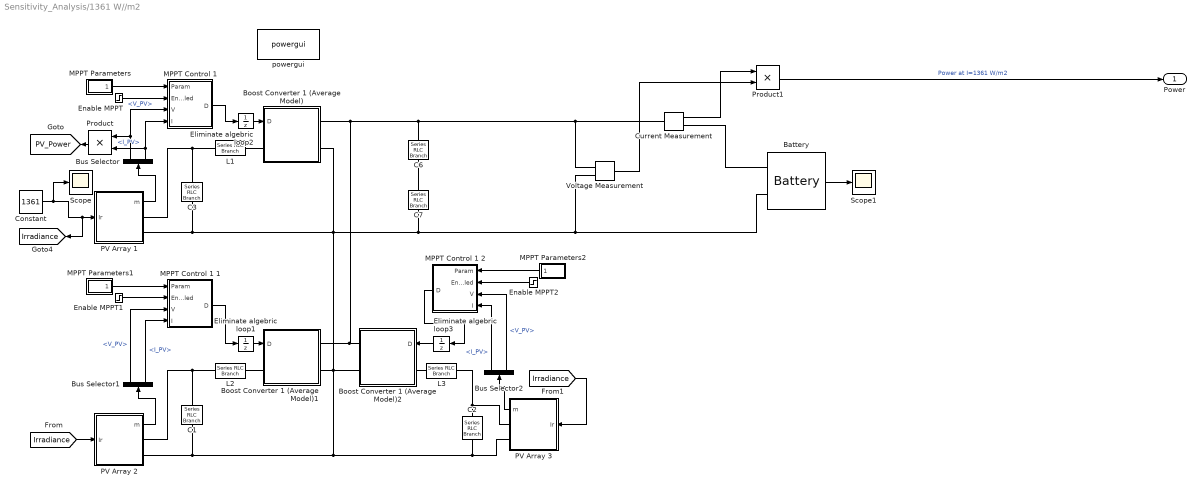
== system Sensitivity_Analysis/1361 W//m2 ==
  Battery : spsBatteryLib/Battery  BatType=Lithium-Ion  ShowTempParam=off  ThermalPreset=no  ShowAgeParam=off  NomV=7.2  NomQ=1000  SOC=100  Batt_Tr=30  PresetModel=on  MaxQ=1000  MinV=5.4  FullV=8.3807  Dis_rate=434.7826  R=7.2e-05  Normal_OP=904.3478  expZone="[7.77878      49.1304]"  current=[6.5 13 32.5]  Units=Time  Tci=20  NomT=20  T2=-30  MaxQ2=4.8  FullV2=7.1  Normal_OP2=5.655  expZone2="[6.58           1]"  Rca=0.6  ti=2000  Dp=0  Neq0=0  Tsim=1e6  Ta1=25  Qeol=5.4*0.9  Reol=0.013333*1.2  Char_age=[2.3478, 3]  Dis_age=[2.3478, 10]  N1=1500  N2=10500  N3=1000  N4=1400  Ta2=45  N5=950
  Boost Converter 1 (Average Model) : Subsystem  mask(Boost Converter (Average Model)){Ts=50e-6}
      mask prompts: Ts "Sample time:"
      mask Display: disp('Boost\n(Average)')
  Boost Converter 1 (Average Model)1 : Subsystem  mask(Boost Converter (Average Model)){Ts=50e-6}
      mask prompts: Ts "Sample time:"
      mask Display: disp('Boost\n(Average)')
  Boost Converter 1 (Average Model)2 : Subsystem  mask(Boost Converter (Average Model)){Ts=50e-6}
      mask prompts: Ts "Sample time:"
      mask Display: disp('Boost\n(Average)')
  Bus Selector : BusSelector  OutputSignals=V_PV,I_PV
  Bus Selector1 : BusSelector  OutputSignals=V_PV,I_PV
  Bus Selector2 : BusSelector  OutputSignals=V_PV,I_PV
  C1 : spsSeriesRLCBranchLib/Series RLC Branch  LConnTagsString=__new0  RConnTagsString=__new0  BranchType=C  Resistance=1.0  Inductance=1.0  SetiL0=off  InitialCurrent=0  Capacitance=100e-6  Setx0=off  InitialVoltage=0  Measurements=Branch voltage
  C2 : spsSeriesRLCBranchLib/Series RLC Branch  LConnTagsString=__new0  RConnTagsString=__new0  BranchType=C  Resistance=1.0  Inductance=1.0  SetiL0=off  InitialCurrent=0  Capacitance=100e-6  Setx0=off  InitialVoltage=0  Measurements=Branch voltage
  C3 : spsSeriesRLCBranchLib/Series RLC Branch  LConnTagsString=__new0  RConnTagsString=__new0  BranchType=C  Resistance=1.0  Inductance=1.0  SetiL0=off  InitialCurrent=0  Capacitance=100e-6  Setx0=off  InitialVoltage=0  Measurements=Branch voltage
  C6 : spsSeriesRLCBranchLib/Series RLC Branch  LConnTagsString=__new0  RConnTagsString=__new0  BranchType=C  Resistance=1.0  Inductance=1.0  SetiL0=off  InitialCurrent=0  Capacitance=24000e-06  Setx0=off  InitialVoltage=0  Measurements=None
  C7 : spsSeriesRLCBranchLib/Series RLC Branch  LConnTagsString=__new0  RConnTagsString=__new0  BranchType=C  Resistance=1.0  Inductance=1.0  SetiL0=off  InitialCurrent=0  Capacitance=24000e-06  Setx0=off  InitialVoltage=0  Measurements=None
  Constant : Constant  Value=1361
  Current Measurement : spsCurrentMeasurementLib/Current Measurement  PhasorSimulation=off  OutputType=Complex  PSBequivalent=0
  Eliminate algebric loop1 : UnitDelay  SampleTime=100e-6  HasFrameUpgradeWarning=on
  Eliminate algebric loop2 : UnitDelay  SampleTime=100e-6  HasFrameUpgradeWarning=on
  Eliminate algebric loop3 : UnitDelay  SampleTime=100e-6  HasFrameUpgradeWarning=on
  Enable MPPT : Step  Time=0.3  SampleTime=0
  Enable MPPT1 : Step  Time=0.3  SampleTime=0
  Enable MPPT2 : Step  Time=0.3  SampleTime=0
  L1 : spsSeriesRLCBranchLib/Series RLC Branch  LConnTagsString=__new0  RConnTagsString=__new0  BranchType=RL  Resistance=0.005  Inductance=5e-3  SetiL0=off  InitialCurrent=0  Capacitance=1e-6  Setx0=off  InitialVoltage=0  Measurements=None
  L2 : spsSeriesRLCBranchLib/Series RLC Branch  LConnTagsString=__new0  RConnTagsString=__new0  BranchType=RL  Resistance=0.005  Inductance=5e-3  SetiL0=off  InitialCurrent=0  Capacitance=1e-6  Setx0=off  InitialVoltage=0  Measurements=None
  L3 : spsSeriesRLCBranchLib/Series RLC Branch  LConnTagsString=__new0  RConnTagsString=__new0  BranchType=RL  Resistance=0.005  Inductance=5e-3  SetiL0=off  InitialCurrent=0  Capacitance=1e-6  Setx0=off  InitialVoltage=0  Measurements=None
  MPPT Parameters : Subsystem
  MPPT Parameters1 : Subsystem
  MPPT Parameters2 : Subsystem
  "MPPT Control 1 " : MATLAB Function  TreatAsAtomicUnit=on
  MPPT Control 1 1 : MATLAB Function  TreatAsAtomicUnit=on
  MPPT Control 1 2 : MATLAB Function  TreatAsAtomicUnit=on
  PV Array 1 : Subsystem  mask(PV array){ModuleType=SunPower SPR-305-WHT, Ncell=96, Nser=2500, Npar=2500, ModuleParameters=[ 64.2  5.96  54.7  5.58 ], ModelParameters=[ 0.037998  993.51  1.1753e-08  5.9602  1.3 ], Ts=50e-6, PlotVI_module=off, PlotVI_array=off}
      mask prompts: ModuleType "Module type:"; Ncell "Number of cells per module"; Nser "Number of series-connected  modules per string"; Npar "Number of parallel strings"; ModuleParameters "Module specifications under STC  [  Voc, Isc, Vmp, Imp ]"; ModelParameters "Model parameters for 1 module [ Rs, Rp, Isat, Iph, Qd ]"; Ts "Sample time"; PlotVI_module "Display  I-V and  P-V characteritics of one module"; PlotVI_array "Display  I-V and  P-V characteritics of array"
      mask help:
      | Model a PV array
      |
      | PV array consists of Npar strings of modules connected in parallel, each string consisting of Nser modules connected in series.
      |
      | The four PV model parameters (photo-generated current Iph, diode saturation current Isat, parallel resistance Rp and  series resistance Rs) are adjuted to fit the following four module characteristics measured under standard test conditions (STC : irradiance 1000 W/m^2, cell temperature=25 deg. C) and assuming a given "diode quality factor" (Qd) for the semiconductor:
      |   Voc = open circuit voltage
      |   Isc = short-circuit current
      |   Vmp,Imp = voltage and current at maximum power point
      |
      | Select a 'Module type' and then press Apply to see module parameters.
      | Note: Module characteristics are extracted from NREL System Advisor Model.
      mask init: same as Sensitivity_Analysis/1000 W//m2/PV Array 1
      mask TypeOptions ModuleType: BP Solar SX3190 | Canadian Solar CS5P-220M | First Solar FS-272 | Kyocera KD135GX-LP | Kyocera KD205GX-LP | Mitsubishi PV-UD190MF5 | Sanyo HIP-225HDE1 | SunPower SPR-305-WHT | SunPower SPR-400-WHT | Suntech STP270S-24_Vb
      mask Display: image(imread('panel.jpg'))
  PV Array 2 : Subsystem  mask(PV array){ModuleType=SunPower SPR-305-WHT, Ncell=96, Nser=2500, Npar=2500, ModuleParameters=[ 64.2  5.96  54.7  5.58 ], ModelParameters=[ 0.037998  993.51  1.1753e-08  5.9602  1.3 ], Ts=50e-6, PlotVI_module=off, PlotVI_array=off}
      mask prompts: ModuleType "Module type:"; Ncell "Number of cells per module"; Nser "Number of series-connected  modules per string"; Npar "Number of parallel strings"; ModuleParameters "Module specifications under STC  [  Voc, Isc, Vmp, Imp ]"; ModelParameters "Model parameters for 1 module [ Rs, Rp, Isat, Iph, Qd ]"; Ts "Sample time"; PlotVI_module "Display  I-V and  P-V characteritics of one module"; PlotVI_array "Display  I-V and  P-V characteritics of array"
      mask help:
      | Model a PV array
      |
      | PV array consists of Npar strings of modules connected in parallel, each string consisting of Nser modules connected in series.
      |
      | The four PV model parameters (photo-generated current Iph, diode saturation current Isat, parallel resistance Rp and  series resistance Rs) are adjuted to fit the following four module characteristics measured under standard test conditions (STC : irradiance 1000 W/m^2, cell temperature=25 deg. C) and assuming a given "diode quality factor" (Qd) for the semiconductor:
      |   Voc = open circuit voltage
      |   Isc = short-circuit current
      |   Vmp,Imp = voltage and current at maximum power point
      |
      | Select a 'Module type' and then press Apply to see module parameters.
      | Note: Module characteristics are extracted from NREL System Advisor Model.
      mask init: same as Sensitivity_Analysis/1000 W//m2/PV Array 1
      mask TypeOptions ModuleType: BP Solar SX3190 | Canadian Solar CS5P-220M | First Solar FS-272 | Kyocera KD135GX-LP | Kyocera KD205GX-LP | Mitsubishi PV-UD190MF5 | Sanyo HIP-225HDE1 | SunPower SPR-305-WHT | SunPower SPR-400-WHT | Suntech STP270S-24_Vb
      mask Display: image(imread('panel.jpg'))
  PV Array 3 : Subsystem  mask(PV array){ModuleType=SunPower SPR-305-WHT, Ncell=96, Nser=2500, Npar=2500, ModuleParameters=[ 64.2  5.96  54.7  5.58 ], ModelParameters=[ 0.037998  993.51  1.1753e-08  5.9602  1.3 ], Ts=50e-6, PlotVI_module=off, PlotVI_array=off}
      mask prompts: ModuleType "Module type:"; Ncell "Number of cells per module"; Nser "Number of series-connected  modules per string"; Npar "Number of parallel strings"; ModuleParameters "Module specifications under STC  [  Voc, Isc, Vmp, Imp ]"; ModelParameters "Model parameters for 1 module [ Rs, Rp, Isat, Iph, Qd ]"; Ts "Sample time"; PlotVI_module "Display  I-V and  P-V characteritics of one module"; PlotVI_array "Display  I-V and  P-V characteritics of array"
      mask help:
      | Model a PV array
      |
      | PV array consists of Npar strings of modules connected in parallel, each string consisting of Nser modules connected in series.
      |
      | The four PV model parameters (photo-generated current Iph, diode saturation current Isat, parallel resistance Rp and  series resistance Rs) are adjuted to fit the following four module characteristics measured under standard test conditions (STC : irradiance 1000 W/m^2, cell temperature=25 deg. C) and assuming a given "diode quality factor" (Qd) for the semiconductor:
      |   Voc = open circuit voltage
      |   Isc = short-circuit current
      |   Vmp,Imp = voltage and current at maximum power point
      |
      | Select a 'Module type' and then press Apply to see module parameters.
      | Note: Module characteristics are extracted from NREL System Advisor Model.
      mask init: same as Sensitivity_Analysis/1000 W//m2/PV Array 1
      mask TypeOptions ModuleType: BP Solar SX3190 | Canadian Solar CS5P-220M | First Solar FS-272 | Kyocera KD135GX-LP | Kyocera KD205GX-LP | Mitsubishi PV-UD190MF5 | Sanyo HIP-225HDE1 | SunPower SPR-305-WHT | SunPower SPR-400-WHT | Suntech STP270S-24_Vb
      mask Display: image(imread('panel.jpg'))
  Product : Product
  Product1 : Product
  Scope : Scope
  Scope1 : Scope
  Voltage Measurement : spsVoltageMeasurementLib/Voltage Measurement  PhasorSimulation=off  OutputType=Complex  PSBequivalent=0
  powergui : sps_lib/powergui  Priority=1  SimulationMode=Continuous  SampleTime=50e-6  frequency=60  Iterations=50  frequencyindice=0  Pbase=100e6  ErrMax=1e-4  UnitsV=kV  UnitsW=MW  buscounter=0  FunctionMessages=off  echomessages=off  EnableUseOfTLC=off  CurrentSourceSwitches=off  DisableSnubberDevices=off  DisableRonSwitches=off  DisableVfSwitches=off  DisplayEquations=off  AutomaticDiscreteSolvers=off  SolverType=Tustin/Backward Euler (TBE)  Interpol=off  ExternalGateDelay=off  methode=off  Ts=100  x0status=blocks  SPID=on  SwTol=0  HookPort=off  NonlinearTolerance=1e-4  nMaxIteration=100  ContinueOnMaxIteration=off  RestoreLinks=warning  ResistiveCurrentMeasurement=off  Frange=[0:2:500]  Ylog=off  Xlog=on  ShowGrid=off  save=off  variable=ZData  structure=0  ZoomFFT=off  StartTime=0.0  cycles=1  DisplayStyle=1  fundamental=60  FreqAxis=off  MaxFrequency=1000  frequencyindicesteady=1  RmsSteady=1  display=off
  Power : Outport
  tag scope: Irradiance=global, PV_Power=global
  wires:
  Voltage Measurement/1 -> Product1/2
  Current Measurement/1 -> Product1/1
  Battery/1 -> Scope1/1
  Eliminate algebric loop2/1 -> Boost Converter 1 (Average Model)/1(D)
  PV Array 2/1(m) -> Bus Selector1/1
  [Irradiance] -> PV Array 3/1(Ir)
  Product/1 -> [PV_Power]
  MPPT Control 1 1/1(D) -> Eliminate algebric loop1/1
  Bus Selector2/1 -> MPPT Control 1 2/3(V)  "<V_PV>"
  Eliminate algebric loop3/1 -> Boost Converter 1 (Average Model)2/1(D)
  MPPT Parameters/1(Param) -> "MPPT Control 1 "/1(Param)
  MPPT Control 1 2/1(D) -> Eliminate algebric loop3/1
  PV Array 3/1(m) -> Bus Selector2/1
  [Irradiance] -> PV Array 2/1(Ir)
  MPPT Parameters1/1(Param) -> MPPT Control 1 1/1(Param)
  Enable MPPT1/1 -> MPPT Control 1 1/2(Enabled)
  Bus Selector/1 -> Product/1, "MPPT Control 1 "/3(V)  "<V_PV>"
  Product1/1 -> Power/1  "Power at I=1361 W/m2"
  "MPPT Control 1 "/1(D) -> Eliminate algebric loop2/1
  MPPT Parameters2/1(Param) -> MPPT Control 1 2/1(Param)
  PV Array 1/1(m) -> Bus Selector/1
  Bus Selector/2 -> Product/2, "MPPT Control 1 "/4(I)  "<I_PV>"
  Bus Selector2/2 -> MPPT Control 1 2/4(I)  "<I_PV>"
  Bus Selector1/2 -> MPPT Control 1 1/4(I)  "<I_PV>"
  Eliminate algebric loop1/1 -> Boost Converter 1 (Average Model)1/1(D)
  Enable MPPT2/1 -> MPPT Control 1 2/2(Enabled)
  Enable MPPT/1 -> "MPPT Control 1 "/2(Enabled)
  Bus Selector1/1 -> MPPT Control 1 1/3(V)  "<V_PV>"
  Constant/1 -> Scope/1, [Irradiance], PV Array 1/1(Ir)
  connections:
  L3/RConn1 -- Boost Converter 1 (Average Model)2/LConn1
  L2/LConn1 -- C1/LConn1 -- PV Array 2/RConn1
  C6/RConn1 -- C7/LConn1
  L2/RConn1 -- Boost Converter 1 (Average Model)1/LConn1
  C3/LConn1 -- L1/LConn1 -- PV Array 1/RConn1
  Battery/LConn2 -- Voltage Measurement/LConn2 -- C2/RConn1 -- PV Array 3/RConn2 -- C1/RConn1 -- PV Array 2/RConn2 -- Boost Converter 1 (Average Model)1/RConn2 -- Boost Converter 1 (Average Model)2/RConn2 -- C3/RConn1 -- PV Array 1/RConn2 -- Boost Converter 1 (Average Model)/RConn2 -- C7/RConn1
  L1/RConn1 -- Boost Converter 1 (Average Model)/LConn1
  Voltage Measurement/LConn1 -- Current Measurement/LConn1 -- Boost Converter 1 (Average Model)1/RConn1 -- Boost Converter 1 (Average Model)2/RConn1 -- Boost Converter 1 (Average Model)/RConn1 -- C6/LConn1
  C2/LConn1 -- L3/LConn1 -- PV Array 3/RConn1
  Current Measurement/RConn1 -- Battery/LConn1
